simulink model "mPowerLossDistributorPassiveCooling"  (R2021b)
settings: Solver=VariableStepAuto  StartTime=0.0  StopTime=10.0  RelTol=1e-3
model workspace (MAT data in the model file):
  AdjacencyMat = [0 0 0 0 0 0 0 0 0 0 0 0 ... (15129 elements, 123x123)]
  CapMat = [1e+20; 2196.70091586; 387.653102799; 193.8265514; 1962.34710525; 387.653102799; 193.8265514; 1962.34710525; 1266.59353814; 268.053957132; 416.539515956; 175.715078; 577.243160678; 310.101557898; 23.9530731873; 15.4990473565; 47.9061463746; 30.998094713; 85.98384; 1.11955442905; 1.11955442905; 1.11955442905; 1.11955442905; 1.11955442905; 1.11955442905; 0.373184809682; 0.373184809682; 450.202206395; 54.9511679003; 54.9511679003; 247.389926005; 247.389926005; 75.306462; 75.306462; 1.11955442905; 1.11955442905; 1e+20; 1e+20; 0; 0; 0; 0; 429.469897824; 0; 0; 0; 0; 429.469897824; 0; 0; 0; 0; 0; 0; 424.408023296; 268.053957132; 0; 0; 0; 0; 0; 322.102423368; 0; 0; 0; 0; 0; 322.102423368; 0; 0; 0; 0; 0; 318.306017472; 268.053957132; 2196.70091586; 1266.59353814; 268.053957132; 416.539515956; 175.715078; 577.243160678; 310.101557898; 85.98384; 0.373184809682; 0.373184809682; 450.202206395; 0; 0; 0; 0; 0; 424.408023296; 268.053957132; 0; 0; 0; 0; 318.306017472; 268.053957132; 2196.70091586; 1266.59353814; 268.053957132; 416.539515956; 175.715078; 577.243160678; 310.101557898; 85.98384; 0.373184809682; 0.373184809682; 450.202206395; 0; 0; 0; 0; 0; 424.408023296; 268.053957132; 0; 0; 0; 0; 318.306017472; 268.053957132]
  CoolantArrayIdxs = [20; 21; 22; 23; 24; 25; 26; 27; 35; 36; 37; 84; 85; 108; 109; 19; 38; 83; 107]
  Friction_Loss_Mat = [0 0 0 0 0 0 0 0 0 0 0 0 ... (2340 elements, 39x60)]
  InletCoolIdxs = [37; 38]
  Iron_Loss_Rotor_Back_Iron_Mat = [0.0117485795538 0.0197051847397 0.0244700561647 0.0255532537599 0.0239976928195 0.0207690118754 0.0168550814705 0.0133554634632 0.01151831468 0.0120080610473 0.0141635691716 0.0169722368466 ... (2340 elements, 39x60)]
  Iron_Loss_Rotor_Pole_Mat = [1.4581490918 1.4537473697 1.43037570585 1.39187577753 1.34319900564 1.28804676124 1.2293784806 1.16971068454 1.11123984852 1.0549546703 0.999931477749 0.94446781724 ... (2340 elements, 39x60)]
  Iron_Loss_Rotor_Tooth_Mat = [0 0 0 0 0 0 0 0 0 0 0 0 ... (2340 elements, 39x60)]
  Iron_Loss_Stator_Back_Iron_Mat = [38.4149877088 37.6503107125 36.6652845221 35.5768425978 34.4225640875 33.2346156756 32.0443324124 30.8866766706 29.801209009 28.7963723188 27.8072961338 26.7363012626 ... (2340 elements, 39x60)]
  Iron_Loss_Stator_Tooth_Mat = [42.0487318978 41.0399202886 40.1567907901 39.4070106899 38.6872815615 37.9480215396 37.175663609 36.3826322946 35.5969122241 34.8195499408 33.9921719085 33.0420249153 ... (2340 elements, 39x60)]
  LossDistrForEachType = [0 0 0 0 0 0 0 0 0 0 0 0 ... (1968 elements, 16x123)]
  Magnet_Loss_Mat = [0.0992355707119 0.0926361497593 0.0866339598393 0.0816717050449 0.0772717421391 0.0730472022398 0.0686189288913 0.0635413555728 0.0572450430654 0.0495346500988 0.0410747136719 0.0327097040848 ... (2340 elements, 39x60)]
  OutletCoolIdxs = [20; 107]
  Rotor_Cage_Loss_Mat = [0 0 0 0 0 0 0 0 0 0 0 0 ... (2340 elements, 39x60)]
  ShaftTorqueVec = [-285.363175319 -270.469371582 -255.575567846 -240.681764109 -225.787960373 -210.894156636 -196.0003529 -181.106549163 -166.212745427 -151.31894169 -136.425137954 -121.531334217 -106.637530481 -91.7437267443 -76.8499230078 -61.9561192713 -47.0623155348 -32.1685117983 -17.2747080618 -2.38090432532 12.5128994112 27.4067031477 42.3005068842 57.1943106207 72.0881143572 86.9819180937 101.87572183 116.769525567 131.663329303 146.55713304 161.450936776 176.344740513 191.238544249 206.132347986 221.026151722 235.919955459 250.813759195 265.707562932 280.601366668]
  SpeedVec = [500 661.016949153 822.033898305 983.050847458 1144.06779661 1305.08474576 1466.10169492 1627.11864407 1788.13559322 1949.15254237 2110.16949153 2271.18644068 2432.20338983 2593.22033898 2754.23728814 2915.25423729 3076.27118644 3237.28813559 3398.30508475 3559.3220339 3720.33898305 3881.3559322 4042.37288136 4203.38983051 4364.40677966 4525.42372881 4686.44067797 4847.45762712 5008.47457627 5169.49152542 5330.50847458 5491.52542373 5652.54237288 5813.55932203 5974.57627119 6135.59322034 6296.61016949 6457.62711864 6618.6440678 6779.66101695 6940.6779661 7101.69491525 7262.71186441 7423.72881356 7584.74576271 7745.76271186 7906.77966102 8067.79661017 8228.81355932 8389.83050847 8550.84745763 8711.86440678 8872.88135593 9033.89830508 9194.91525424 9355.93220339 9516.94915254 9677.96610169 9838.98305085 10000]
  StateSpaceND : object (value not decoded)
  StatorCopperTempCoefResistivity = 0.00393
  Stator_Copper_Loss_Mat = [4036.39837515 3610.67609702 3178.68722837 2791.06956208 2441.07338047 2123.72912642 1835.28722535 1572.85477291 1334.16141597 1117.77314243 921.650266023 744.483696972 ... (2340 elements, 39x60)]
  Stray_Load_Loss_Mat = [0 0 0 0 0 0 0 0 0 0 0 0 ... (2340 elements, 39x60)]
  Stray_Loss_Stator_Iron_Proportion = 0.95
  Tgiven = 20
  TnodesInit = [25; 25; 25; 25; 25; 25; 25; 25; 25; 25; 25; 25; 25; 25; 25; 25; 25; 25; 25; 25; 25; 25; 25; 25; 25; 25; 25; 25; 25; 25; 25; 25; 25; 25; 25; 25; 25; 25; 25; 25; 25; 25; 25; 25; 25; 25; 25; 25; 25; 25; 25; 25; 25; 25; 25; 25; 25; 25; 25; 25; 25; 25; 25; 25; 25; 25; 25; 25; 25; 25; 25; 25; 25; 25; 25; 25; 25; 25; 25; 25; 25; 25; 25; 25; 25; 25; 25; 25; 25; 25; 25; 25; 25; 25; 25; 25; 25; 25; 25; 25; 25; 25; 25; 25; 25; 25; 25; 25; 25; 25; 25; 25; 25; 25; 25; 25; 25; 25; 25; 25; 25; 25; 25]
  Tsim = 20
  Windage_Loss_Mat = [0 0 0 0 0 0 0 0 0 0 0 0 ... (2340 elements, 39x60)]
  armatureCopperLossVal = 35
  backIronLossVal = 15
  magnetLossVal = 12
  speedVal = 2000
  toothIronLossVal = 25
  torqueVal = 20
libraries: mcadROM_lib x2
(part 1 of 2)
settings Model: Creator=agonzale  LastModifiedBy=agonzale

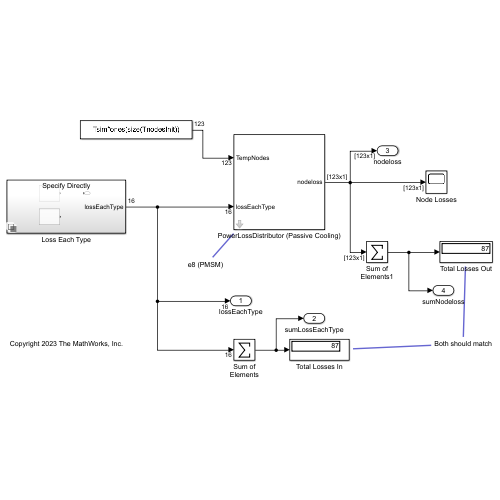
[thumbnail: Simulink's stored preview of the top-level diagram]
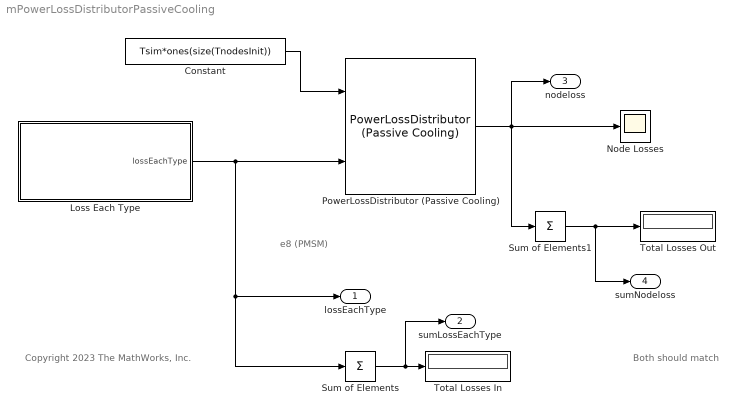
== system mPowerLossDistributorPassiveCooling ==
  note: e8 (PMSM)
  note: Both should match
  note: Copyright 2023 The MathWorks, Inc.
  Constant : Constant  Value=Tsim*ones(size(TnodesInit))
  Loss Each Type : Subsystem  Variant=on  VariantControlMode=label  VariantControl=Choice  LabelModeActiveChoice=Specify Directly
  Node Losses : Scope
  PowerLossDistributor (Passive Cooling) : mcadROM_lib/PowerLossDistributor (Passive Cooling)  TrefStator=20  StatorCopperTempCoefResistivity=StatorCopperTempCoefResistivity  TrefRotor=20  RotorCopperTempCoefResistivity=1e-5  LossDistrForEachType=LossDistrForEachType  CapMat=CapMat
  Sum of Elements : Sum  Inputs=+
  Sum of Elements1 : Sum  Inputs=+
  Total Losses In : Display
  Total Losses Out : Display
  lossEachType : Outport
  sumLossEachType : Outport  Port=2
  nodeloss : Outport  Port=3  PortDimensions=[123,1]
  sumNodeloss : Outport  Port=4
  wires:
  Sum of Elements/1 -> sumLossEachType/1, Total Losses In/1
  Constant/1 -> PowerLossDistributor (Passive Cooling)/1
  Loss Each Type/1(lossEachType) -> PowerLossDistributor (Passive Cooling)/2, Sum of Elements/1, lossEachType/1
  Sum of Elements1/1 -> sumNodeloss/1, Total Losses Out/1
  PowerLossDistributor (Passive Cooling)/1 -> Sum of Elements1/1, Node Losses/1, nodeloss/1
